simulink model "Mirror_Subsystem"  (R2018a)
settings: Solver=VariableStepAuto  StartTime=0.0  StopTime=10.0  RelTol=1e-3
settings Model: Creator=99003191  LastModifiedBy=Anoosha Clarance
settings DataIOCC: ReturnWorkspaceOutputs=on
settings SFSimCC: SimUseLocalCustomCode=on
settings RTWCC: RTWUseLocalCustomCode=on

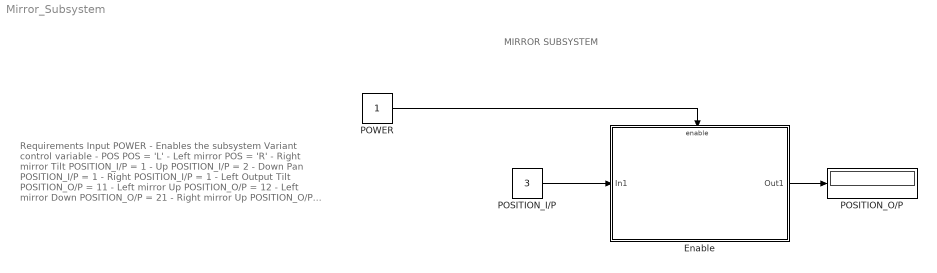
== system Mirror_Subsystem ==
  note: Requirements
      | Input
      | POWER - Enables the subsystem
      | Variant control variable - POS
      | POS = 'L' - Left mirror
      | POS = 'R' - Right mirror
      | Tilt
      | POSITION_I/P = 1 - Up
      | POSITION_I/P = 2 - Down
      | Pan
      | POSITION_I/P = 1 - Right
      | POSITION_I/P = 1 - Left
      |
      | Output
      | Tilt
      | POSITION_O/P = 11 - Left mirror Up
      | POSITION_O/P = 12 - Left mirror Down
      | POSITION_O/P = 21 - Right mirror Up
      | POSITION_O/P = 22 - Right mirror Down
      | Pan
      | POSITION_O/P = 13 - Left mirror Right
      | POSITION_O/P = 14 - Left mirror Left
      | POSITION_O/P = 23 - Right mirror Right
      | POSITION_O/P = 24 - Right mirror Left
  note: MIRROR SUBSYSTEM
  Enable : Subsystem  TreatAsAtomicUnit=on
  POSITION_I/P : Constant  Value=3
  POSITION_O/P : Display
  POWER : Constant
  wires:
  Enable/1(Out1) -> POSITION_O/P/1
  POSITION_I/P/1 -> Enable/1(In1)
  POWER/1 -> Enable/Enable

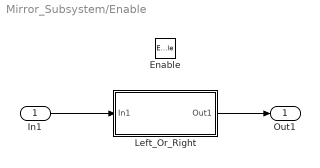
== system Mirror_Subsystem/Enable ==
  In1 : Inport
  Enable : EnablePort
  Left_Or_Right : Subsystem  Variant=on
  Out1 : Outport
  wires:
  In1/1 -> Left_Or_Right/1(In1)
  Left_Or_Right/1(Out1) -> Out1/1

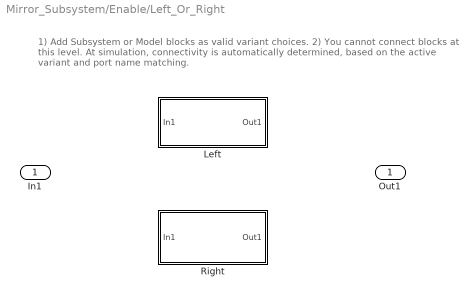
== system Mirror_Subsystem/Enable/Left_Or_Right ==
  note: 1) Add Subsystem or Model blocks as valid variant choices.
      | 2) You cannot connect blocks at this level. At simulation, connectivity is automatically
      | determined, based on the active variant and port name matching.
  In1 : Inport
  Left : Subsystem  VariantControl=POS == 'L'
  Right : Subsystem  VariantControl=POS == 'R'
  Out1 : Outport

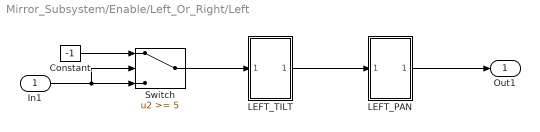
== system Mirror_Subsystem/Enable/Left_Or_Right/Left ==
  In1 : Inport
  Constant : Constant  Value=-1
  LEFT_PAN : Subsystem
  LEFT_TILT : Subsystem
  Switch : Switch  Threshold=5
  Out1 : Outport
  wires:
  In1/1 -> Switch/2, Switch/3
  Constant/1 -> Switch/1
  Switch/1 -> LEFT_TILT/1(In1)
  LEFT_TILT/1(Out1) -> LEFT_PAN/1(In1)
  LEFT_PAN/1(Out1) -> Out1/1

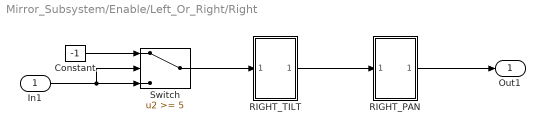
== system Mirror_Subsystem/Enable/Left_Or_Right/Right ==
  In1 : Inport
  Constant : Constant  Value=-1
  RIGHT_PAN : Subsystem
  RIGHT_TILT : Subsystem
  Switch : Switch  Threshold=5
  Out1 : Outport
  wires:
  Constant/1 -> Switch/1
  RIGHT_PAN/1(Out1) -> Out1/1
  Switch/1 -> RIGHT_TILT/1(In1)
  In1/1 -> Switch/2, Switch/3
  RIGHT_TILT/1(Out1) -> RIGHT_PAN/1(In1)

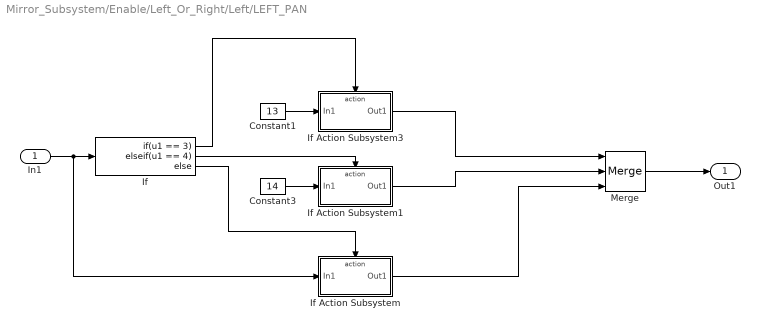
== system Mirror_Subsystem/Enable/Left_Or_Right/Left/LEFT_PAN ==
  In1 : Inport
  Constant1 : Constant  Value=13
  Constant3 : Constant  Value=14
  If : If  IfExpression=u1 == 3  ElseIfExpressions=u1 == 4
  If Action Subsystem : Subsystem  TreatAsAtomicUnit=on
  If Action Subsystem1 : Subsystem  TreatAsAtomicUnit=on
  If Action Subsystem3 : Subsystem  TreatAsAtomicUnit=on
  Merge : Merge  Inputs=3
  Out1 : Outport
  wires:
  Constant1/1 -> If Action Subsystem3/1(In1)
  If/1 -> If Action Subsystem3/Action
  Merge/1 -> Out1/1
  If/2 -> If Action Subsystem1/Action
  Constant3/1 -> If Action Subsystem1/1(In1)
  If Action Subsystem3/1(Out1) -> Merge/1
  If Action Subsystem1/1(Out1) -> Merge/2
  If/3 -> If Action Subsystem/Action
  In1/1 -> If Action Subsystem/1(In1), If/1
  If Action Subsystem/1(Out1) -> Merge/3

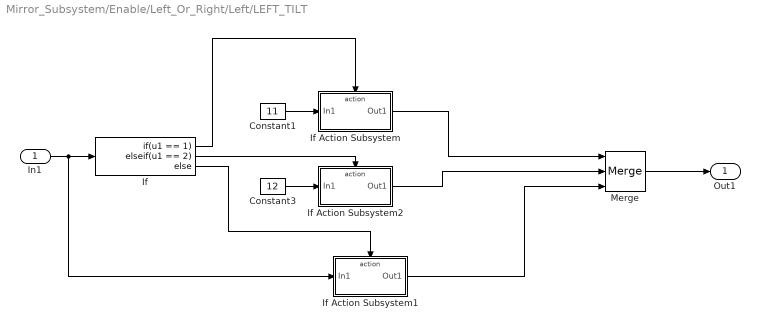
== system Mirror_Subsystem/Enable/Left_Or_Right/Left/LEFT_TILT ==
  In1 : Inport
  Constant1 : Constant  Value=11
  Constant3 : Constant  Value=12
  If : If  IfExpression=u1 == 1  ElseIfExpressions=u1 == 2
  If Action Subsystem : Subsystem  TreatAsAtomicUnit=on
  If Action Subsystem1 : Subsystem  TreatAsAtomicUnit=on
  If Action Subsystem2 : Subsystem  TreatAsAtomicUnit=on
  Merge : Merge  Inputs=3
  Out1 : Outport
  wires:
  If/2 -> If Action Subsystem2/Action
  If/1 -> If Action Subsystem/Action
  Constant1/1 -> If Action Subsystem/1(In1)
  If Action Subsystem/1(Out1) -> Merge/1
  Merge/1 -> Out1/1
  If Action Subsystem2/1(Out1) -> Merge/2
  Constant3/1 -> If Action Subsystem2/1(In1)
  If/3 -> If Action Subsystem1/Action
  If Action Subsystem1/1(Out1) -> Merge/3
  In1/1 -> If Action Subsystem1/1(In1), If/1

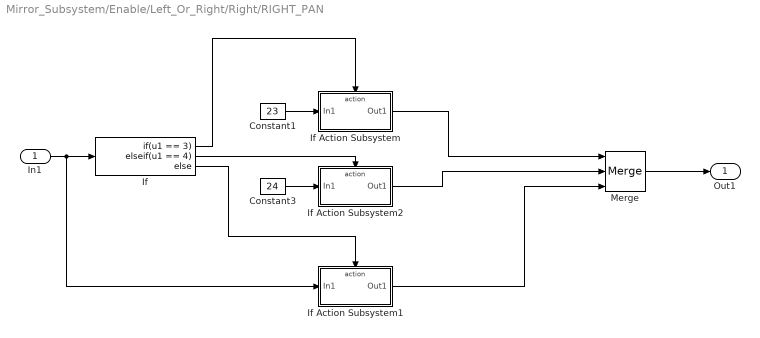
== system Mirror_Subsystem/Enable/Left_Or_Right/Right/RIGHT_PAN ==
  In1 : Inport
  Constant1 : Constant  Value=23
  Constant3 : Constant  Value=24
  If : If  IfExpression=u1 == 3  ElseIfExpressions=u1 == 4
  If Action Subsystem : Subsystem  TreatAsAtomicUnit=on
  If Action Subsystem1 : Subsystem  TreatAsAtomicUnit=on
  If Action Subsystem2 : Subsystem  TreatAsAtomicUnit=on
  Merge : Merge  Inputs=3
  Out1 : Outport
  wires:
  Constant1/1 -> If Action Subsystem/1(In1)
  If/1 -> If Action Subsystem/Action
  Merge/1 -> Out1/1
  If/2 -> If Action Subsystem2/Action
  Constant3/1 -> If Action Subsystem2/1(In1)
  If Action Subsystem/1(Out1) -> Merge/1
  If Action Subsystem2/1(Out1) -> Merge/2
  In1/1 -> If Action Subsystem1/1(In1), If/1
  If/3 -> If Action Subsystem1/Action
  If Action Subsystem1/1(Out1) -> Merge/3

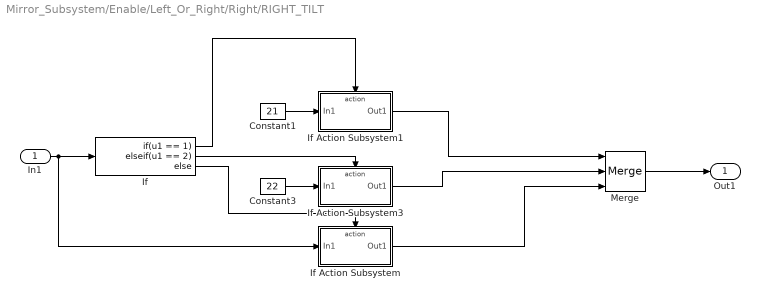
== system Mirror_Subsystem/Enable/Left_Or_Right/Right/RIGHT_TILT ==
  In1 : Inport
  Constant1 : Constant  Value=21
  Constant3 : Constant  Value=22
  If : If  IfExpression=u1 == 1  ElseIfExpressions=u1 == 2
  If Action Subsystem : Subsystem  TreatAsAtomicUnit=on
  If Action Subsystem1 : Subsystem  TreatAsAtomicUnit=on
  If Action Subsystem3 : Subsystem  TreatAsAtomicUnit=on
  Merge : Merge  Inputs=3
  Out1 : Outport
  wires:
  If/2 -> If Action Subsystem3/Action
  If/1 -> If Action Subsystem1/Action
  Constant1/1 -> If Action Subsystem1/1(In1)
  If Action Subsystem1/1(Out1) -> Merge/1
  Merge/1 -> Out1/1
  If Action Subsystem3/1(Out1) -> Merge/2
  In1/1 -> If Action Subsystem/1(In1), If/1
  Constant3/1 -> If Action Subsystem3/1(In1)
  If/3 -> If Action Subsystem/Action
  If Action Subsystem/1(Out1) -> Merge/3

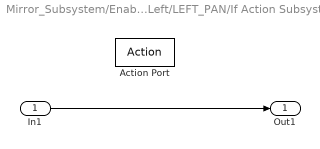
== system Mirror_Subsystem/Enable/Left_Or_Right/Left/LEFT_PAN/If Action Subsystem ==
  In1 : Inport
  Action Port : ActionPort
  Out1 : Outport
  wires:
  In1/1 -> Out1/1

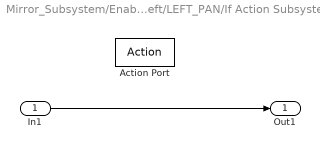
== system Mirror_Subsystem/Enable/Left_Or_Right/Left/LEFT_PAN/If Action Subsystem1 ==
  In1 : Inport
  Action Port : ActionPort
  Out1 : Outport
  wires:
  In1/1 -> Out1/1

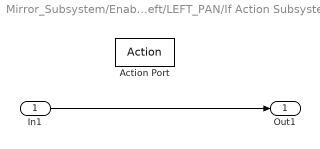
== system Mirror_Subsystem/Enable/Left_Or_Right/Left/LEFT_PAN/If Action Subsystem3 ==
  In1 : Inport
  Action Port : ActionPort
  Out1 : Outport
  wires:
  In1/1 -> Out1/1

== system Mirror_Subsystem/Enable/Left_Or_Right/Left/LEFT_TILT/If Action Subsystem ==
  In1 : Inport
  Action Port : ActionPort
  Out1 : Outport
  wires:
  In1/1 -> Out1/1

== system Mirror_Subsystem/Enable/Left_Or_Right/Left/LEFT_TILT/If Action Subsystem1 ==
  In1 : Inport
  Action Port : ActionPort
  Out1 : Outport
  wires:
  In1/1 -> Out1/1

== system Mirror_Subsystem/Enable/Left_Or_Right/Left/LEFT_TILT/If Action Subsystem2 ==
  In1 : Inport
  Action Port : ActionPort
  Out1 : Outport
  wires:
  In1/1 -> Out1/1

== system Mirror_Subsystem/Enable/Left_Or_Right/Right/RIGHT_PAN/If Action Subsystem ==
  In1 : Inport
  Action Port : ActionPort
  Out1 : Outport
  wires:
  In1/1 -> Out1/1

== system Mirror_Subsystem/Enable/Left_Or_Right/Right/RIGHT_PAN/If Action Subsystem1 ==
  In1 : Inport
  Action Port : ActionPort
  Out1 : Outport
  wires:
  In1/1 -> Out1/1

== system Mirror_Subsystem/Enable/Left_Or_Right/Right/RIGHT_PAN/If Action Subsystem2 ==
  In1 : Inport
  Action Port : ActionPort
  Out1 : Outport
  wires:
  In1/1 -> Out1/1

== system Mirror_Subsystem/Enable/Left_Or_Right/Right/RIGHT_TILT/If Action Subsystem ==
  In1 : Inport
  Action Port : ActionPort
  Out1 : Outport
  wires:
  In1/1 -> Out1/1

== system Mirror_Subsystem/Enable/Left_Or_Right/Right/RIGHT_TILT/If Action Subsystem1 ==
  In1 : Inport
  Action Port : ActionPort
  Out1 : Outport
  wires:
  In1/1 -> Out1/1

== system Mirror_Subsystem/Enable/Left_Or_Right/Right/RIGHT_TILT/If Action Subsystem3 ==
  In1 : Inport
  Action Port : ActionPort
  Out1 : Outport
  wires:
  In1/1 -> Out1/1
